simulink model "Lyapunov_method_implementation"  (R2025b)
settings: Solver=VariableStepAuto  StartTime=0.0  StopTime=4  RelTol=1e-3
settings Model: Creator=lucag  LastModifiedBy=lucag

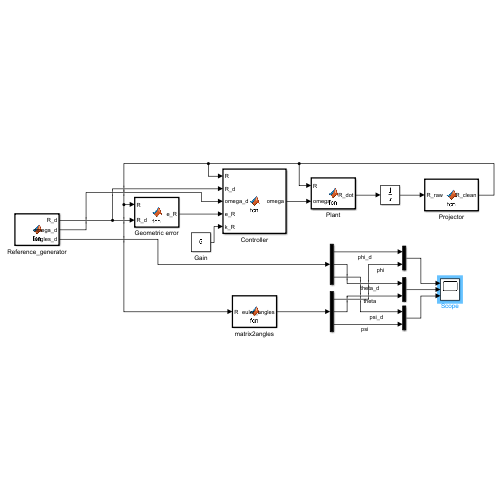
[thumbnail: Simulink's stored preview of the top-level diagram]
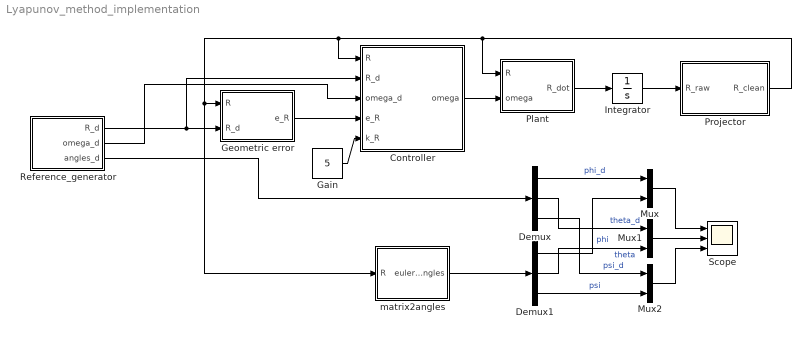
== system Lyapunov_method_implementation ==
  Controller : MATLAB Function  TreatAsAtomicUnit=on
  Demux : Demux  Outputs=3
  Demux1 : Demux  Outputs=3
  Gain : Constant  Value=5
  Geometric error : MATLAB Function  TreatAsAtomicUnit=on
  Integrator : Integrator  InitialCondition=eye(3)
  Mux : Mux  Inputs=2
  Mux1 : Mux  Inputs=2
  Mux2 : Mux  Inputs=2
  Plant : MATLAB Function  TreatAsAtomicUnit=on
  Projector : MATLAB Function  TreatAsAtomicUnit=on
  Reference_generator : MATLAB Function  TreatAsAtomicUnit=on
  Scope : Scope  NumInputPorts=3
      settings: ActiveDisplayYMinimum=-0.098174770424681007  ActiveDisplayYMaximum=0.88357293382212931
  matrix2angles : MATLAB Function  TreatAsAtomicUnit=on
  wires:
  Plant/1(R_dot) -> Integrator/1
  Controller/1(omega) -> Plant/2(omega)
  Geometric error/1(e_R) -> Controller/4(e_R)
  Gain/1 -> Controller/5(k_R)
  Reference_generator/1(R_d) -> Controller/2(R_d), Geometric error/2(R_d)
  Reference_generator/2(omega_d) -> Controller/3(omega_d)
  Projector/1(R_clean) -> Controller/1(R), matrix2angles/1(R), Geometric error/1(R), Plant/1(R)
  Integrator/1 -> Projector/1(R_raw)
  Reference_generator/3(angles_d) -> Demux/1
  matrix2angles/1(euler_angles) -> Demux1/1
  Demux/1 -> Mux/1  "phi_d"
  Demux1/1 -> Mux/2  "phi"
  Demux/2 -> Mux1/1  "theta_d"
  Demux1/2 -> Mux1/2  "theta"
  Demux/3 -> Mux2/1  "psi_d"
  Demux1/3 -> Mux2/2  "psi"
  Mux/1 -> Scope/1
  Mux1/1 -> Scope/2
  Mux2/1 -> Scope/3

== matlab function Lyapunov_method_implementation/Controller ==
  data: R input; omega output; R_d input; omega_d input; e_R input; k_R input
function omega = fcn(R, R_d, omega_d, e_R, k_R)
    % Feedforward term rotated into current body frame
    feedforward = R' * R_d * omega_d;

    % Proportional feedback term
    feedback = -k_R * e_R;

    % Total control effort
    omega = feedforward + feedback;
end

== matlab function Lyapunov_method_implementation/Geometric error ==
  data: R input; e_R output; R_d input
function e_R = fcn(R, R_d)
    % Calculate the skew-symmetric error matrix
    S = 0.5 * (R_d' * R - R' * R_d);

    % Apply the vee map to extract the vector
    e_R = [S(3,2); S(1,3); S(2,1)];
end

== matlab function Lyapunov_method_implementation/Plant ==
  data: R input; R_dot output; omega input
function R_dot = fcn(R, omega)
    % Apply the hat map to omega
    omega_hat = [   0,      -omega(3),  omega(2);
                 omega(3),      0,     -omega(1);
                -omega(2),  omega(1),      0    ];

    % Bilinear differential equation
    R_dot = R * omega_hat;
end

== matlab function Lyapunov_method_implementation/Reference_generator ==
  data: R_d output; omega_d output; angles_d output
function [R_d, omega_d, angles_d] = fcn()
% For now generate constant reference matrix R_d using fixes Roll
% (phi), Pitch (theta) and Yaw (psi) angles
phi = pi/4;
theta = pi/4;
psi = pi/4;

angles_d = [phi, theta, psi];

R11 = cos(psi)*cos(theta);
R12 = cos(psi)*sin(theta)*sin(phi) - sin(psi)*cos(phi);
R13 = cos(psi)*sin(theta)*cos(phi) + sin(psi)*sin(phi);
R21 = sin(psi)*cos(theta);
R22 = sin(psi)*sin(theta)*sin(phi) + cos(psi)*cos(phi);
R23 = sin(psi)*sin(theta)*cos(phi) - cos(psi)*sin(phi);
R31 = -sin(theta);
R32 = cos(theta)*sin(phi);
R33 = cos(theta)*cos(phi);

R_d = [R11 R12 R13;
    R21 R22 R23;
    R31 R32 R33];

% For now generate constand reference
omega_d = [0,0,0]';
end

== matlab function Lyapunov_method_implementation/Projector ==
  data: R_raw input; R_clean output
function R_clean = fcn(R_raw)
    % This script is used to project back on SO(3) the output of the
    % integrator, which can no longer be a valid rotation matrix due to
    % numerical intgration errors.

    % Perform SVD
    [U, ~, V] = svd(R_raw);
    
    % Reconstruct the closest orthogonal matrix
    R_clean = U * V';
    
    % Ensure determinant is +1 (proper rotation, not reflection)
    if det(R_clean) < 0
        U(:,3) = -U(:,3);
        R_clean = U * V';
    end
end

== matlab function Lyapunov_method_implementation/matrix2angles ==
  data: euler_angles output; R input
function euler_angles = fcn(R)
    % Extracts 3-2-1 (Yaw-Pitch-Roll) Euler angles from a Rotation Matrix
    % Output: euler_angles = [Roll (phi); Pitch (theta); Yaw (psi)] in radians

    % Extract matrix elements for readability
    r11 = R(1,1);
    r21 = R(2,1);
    r31 = R(3,1);
    r32 = R(3,2);
    r33 = R(3,3);

    % Roll (phi) - rotation about body X axis
    phi = atan2(r32, r33);

    % Pitch (theta) - rotation about body Y axis
    % Note: Using atan2 with the square root instead of asin(-r31) prevents 
    % Simulink from throwing complex number errors due to floating point drift
    theta = atan2(-r31, sqrt(r32^2 + r33^2));

    % Yaw (psi) - rotation about body Z axis
    psi = atan2(r21, r11);

    % Pack into a 3x1 column vector
    euler_angles = [phi; theta; psi];
end
